simulink model "modelWithControllerAndBasicRobotDynamics"  (R2022a)
settings: Solver=VariableStepAuto  StartTime=0.0  StopTime=20  MaxStep=0.1  RelTol=1e-2  AbsTol=1e-2
model workspace (MAT data in the model file):
  jointLimits = [-2.94087978961  2.94087978961; -2.50454747661  0.759218224618; -2.94087978961  2.94087978961; -2.15548162621  1.3962634016; -5.06145483078  5.06145483078; -1.53588974176  2.40855436775; -3.99680398707  3.99680398707; 0  0.025; 0  0.025; -2.94087978961  2.94087978961; -2.50454747661  0.759218224618; -2.94087978961  2.94087978961; -2.15548162621  1.3962634016; -5.06145483078  5.06145483078; -1.53588974176  2.40855436775; -3.99680398707  3.99680398707; 0  0.025; 0  0.025]
values from neighbouring files (symbols this model uses):
  configSequence = [-0.501061022402 -0.485319444061 0.447530394494 -0.0261030910079 -0.440724306093 0.594332377665 0.0114553342542 0 0 0.712315437264 -1.59156502907 -0.483414164072 ... (126 elements, 18x7)]    [abbExampleRSTVariables.mat]    (also in abbSavedConfigs.mat)
  dq0 = [0 0 0 0 0 0 0 0 0 0 0 0 ... (18 elements, 18x1)]    [abbExampleRSTVariables.mat]
  q0 = [-0.501061022402 -0.485319444061 0.447530394494 -0.0261030910079 -0.440724306093 0.594332377665 0.0114553342542 0 0 0.712315437264 -1.59156502907 -0.483414164072 ... (18 elements, 18x1)]    [abbExampleRSTVariables.mat]
undefined symbols (not defined in the file or in its folder): robot
libraries: robotmaniplib x4, robotcorelib x1
settings Model: PauseTimes=3.1  Creator=The MathWorks, Inc.  LastModifiedBy=The MathWorks, Inc.
settings SolverCC: AlgebraicLoopSolver=TrustRegion
settings DebuggingCC: UnconnectedInputMsg=warning  UnconnectedOutputMsg=warning  UnconnectedLineMsg=warning  SFMachineParentedDataDiag=warning

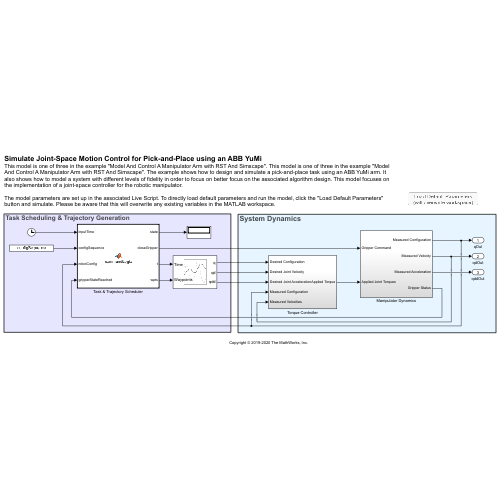
[thumbnail: Simulink's stored preview of the top-level diagram]
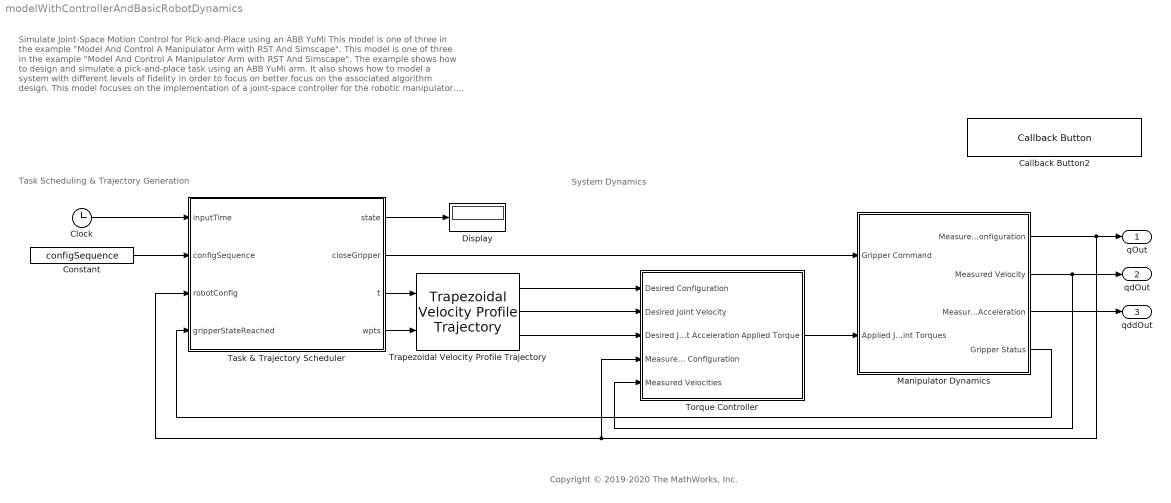
== system modelWithControllerAndBasicRobotDynamics ==
  note: Task Scheduling & Trajectory Generation
  note: System Dynamics
  note: Copyright © 2019-2020 The MathWorks, Inc.
  note: Simulate Joint-Space Motion Control for Pick-and-Place using an ABB YuMi
      | This model is one of three in the example "Model And Control A Manipulator Arm with RST And Simscape". This model is one of three in the example "Model And Control A Manipulator Arm with RST And Simscape". The example shows how to design and simulate a pick-and-place task using an ABB YuMi arm. It also shows how to model a system with different levels of fidelity in order to focus on better focus on the associated algorithm design. This model focuses on the implementation of a joint-space controller for the robotic manipulator.
      |
      | The model parameters are set up in the associated Live Script. To directly load default parameters and run the model, click the "Load Default Parameters" button and simulate. Please be aware that this will overwrite any existing variables in the MATLAB workspace.
  Callback Button2 : CallbackButton  ButtonText=Load Default Parameters (will overwrite workspace)
      settings: ClickFcn=|
      | robot = loadrobot('abbYumi', 'Gravity', [0 0 -9.81]);
      | load abbExampleRSTVariables.mat;
  Clock : Clock
  Constant : Constant  Value=configSequence
  Display : Display
  Manipulator Dynamics : Subsystem
  Task & Trajectory Scheduler : MATLAB Function  TreatAsAtomicUnit=on
  Torque Controller : Subsystem
  Trapezoidal Velocity Profile Trajectory : robotcorelib/Trapezoidal Velocity Profile Trajectory  WaypointSource=External  Waypoints=[ 0, -0.5, -1; 0, 0.5, 1 ]  NumParams=1  Parameter1=End Time  Parameter2=End Time  ParameterSource=Internal  PeakVelocity=[ 2; 2 ]  Acceleration=[ 1; 2 ]  EndTime=2  AccelTime=[ 1; 2 ]  SimulateUsing=Interpreted execution
      settings: SourceProductBaseCode=RO,NV,RR,UV
  qOut : Outport
  qdOut : Outport  Port=2
  qddOut : Outport  Port=3
  wires:
  Task & Trajectory Scheduler/3(t) -> Trapezoidal Velocity Profile Trajectory/1
  Task & Trajectory Scheduler/4(wpts) -> Trapezoidal Velocity Profile Trajectory/2
  Constant/1 -> Task & Trajectory Scheduler/2(configSequence)
  Task & Trajectory Scheduler/1(state) -> Display/1
  Trapezoidal Velocity Profile Trajectory/1 -> Torque Controller/1(Desired Configuration)
  Trapezoidal Velocity Profile Trajectory/2 -> Torque Controller/2(Desired Joint Velocity)
  Trapezoidal Velocity Profile Trajectory/3 -> Torque Controller/3(Desired Joint Acceleration)
  Manipulator Dynamics/1(Measured Configuration) -> Torque Controller/4(Measured Configuration), Task & Trajectory Scheduler/3(robotConfig), qOut/1
  Manipulator Dynamics/2(Measured Velocity) -> Torque Controller/5(Measured Velocities), qdOut/1
  Manipulator Dynamics/3(Measured Acceleration) -> qddOut/1
  Manipulator Dynamics/4(Gripper Status) -> Task & Trajectory Scheduler/4(gripperStateReached)
  Torque Controller/1(Applied Torque) -> Manipulator Dynamics/2(Applied Joint Torques)
  Task & Trajectory Scheduler/2(closeGripper) -> Manipulator Dynamics/1(Gripper Command)
  Clock/1 -> Task & Trajectory Scheduler/1(inputTime)

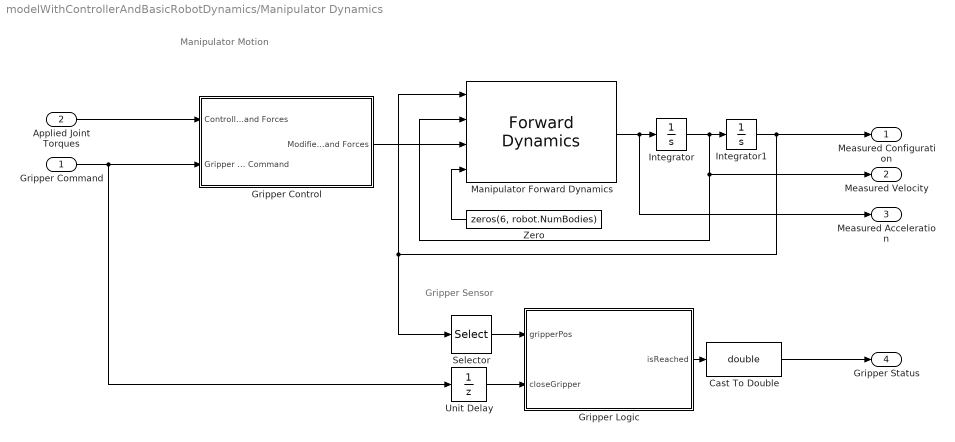
== system modelWithControllerAndBasicRobotDynamics/Manipulator Dynamics ==
  note: Gripper Sensor
  note: Manipulator Motion
  Gripper Command : Inport
  Applied Joint Torques : Inport  Port=2
  Cast To Double : DataTypeConversion  OutDataTypeStr=double  SaturateOnIntegerOverflow=off  RndMeth=Floor
  Gripper Control : Subsystem
  Gripper Logic : MATLAB Function  TreatAsAtomicUnit=on
  Integrator : Integrator  InitialCondition=dq0
  Integrator1 : Integrator  InitialCondition=q0  LimitOutput=on  UpperSaturationLimit=jointLimits(:,2)  LowerSaturationLimit=jointLimits(:,1)
  Manipulator Forward Dynamics : robotmaniplib/Forward Dynamics  RigidBodyTree=robot  SimulateUsing=Interpreted execution
  Selector : Selector  InputPortWidth=18  IndexOptions=Index vector (dialog)  Indices=[17 18]  OutputSizes=1
  Unit Delay : UnitDelay  SampleTime=-1  HasFrameUpgradeWarning=on
  Zero : Constant  Value=zeros(6, robot.NumBodies)  OutDataTypeStr=Inherit: Inherit via back propagation
  Measured Configuration : Outport  VectorParamsAs1DForOutWhenUnconnected=off
  Measured Velocity : Outport  Port=2  VectorParamsAs1DForOutWhenUnconnected=off
  Measured Acceleration : Outport  Port=3  VectorParamsAs1DForOutWhenUnconnected=off
  Gripper Status : Outport  Port=4  VectorParamsAs1DForOutWhenUnconnected=off
  wires:
  Zero/1 -> Manipulator Forward Dynamics/4
  Applied Joint Torques/1 -> Gripper Control/1(Controller Joint Torques and Forces)
  Integrator/1 -> Manipulator Forward Dynamics/2, Measured Velocity/1, Integrator1/1
  Manipulator Forward Dynamics/1 -> Integrator/1, Measured Acceleration/1
  Gripper Command/1 -> Unit Delay/1, Gripper Control/2(Gripper Close Command)
  Gripper Control/1(Modified Joint Torques and Forces) -> Manipulator Forward Dynamics/3
  Selector/1 -> Gripper Logic/1(gripperPos)
  Gripper Logic/1(isReached) -> Cast To Double/1
  Cast To Double/1 -> Gripper Status/1
  Unit Delay/1 -> Gripper Logic/2(closeGripper)
  Integrator1/1 -> Selector/1, Manipulator Forward Dynamics/1, Measured Configuration/1

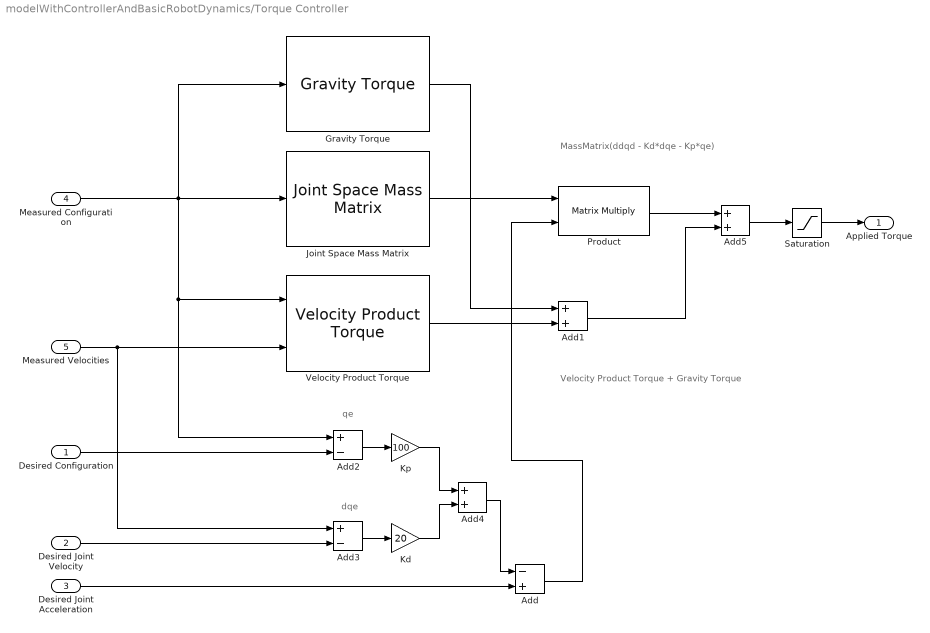
== system modelWithControllerAndBasicRobotDynamics/Torque Controller ==
  note: MassMatrix(ddqd - Kd*dqe - Kp*qe)
  note: Velocity Product Torque + Gravity Torque
  note: dqe
  note: qe
  Desired Configuration : Inport
  Desired Joint Velocity : Inport  Port=2
  Desired Joint Acceleration : Inport  Port=3
  Measured Configuration : Inport  Port=4
  Measured Velocities : Inport  Port=5
  Add : Sum  Inputs=-+
  Add1 : Sum
  Add2 : Sum  Inputs=+-
  Add3 : Sum  Inputs=+-
  Add4 : Sum
  Add5 : Sum
  Gravity Torque : robotmaniplib/Gravity Torque  RigidBodyTree=robot  SimulateUsing=Interpreted execution
  Joint Space Mass Matrix : robotmaniplib/Joint Space Mass Matrix  RigidBodyTree=robot  SimulateUsing=Interpreted execution
  Kd : Gain  Gain=20
  Kp : Gain  Gain=100
  Product : Product  Multiplication=Matrix(*)
  Saturation : Saturate  UpperLimit=100  LowerLimit=-100
  Velocity Product Torque : robotmaniplib/Velocity Product Torque  RigidBodyTree=robot  SimulateUsing=Interpreted execution
      settings: SourceProductBaseCode=RO
  Applied Torque : Outport  VectorParamsAs1DForOutWhenUnconnected=off
  wires:
  Saturation/1 -> Applied Torque/1
  Velocity Product Torque/1 -> Add1/2
  Gravity Torque/1 -> Add1/1
  Add1/1 -> Add5/2
  Product/1 -> Add5/1
  Add5/1 -> Saturation/1
  Kd/1 -> Add4/2
  Kp/1 -> Add4/1
  Add3/1 -> Kd/1
  Add2/1 -> Kp/1
  Add/1 -> Product/2
  Add4/1 -> Add/1
  Measured Velocities/1 -> Velocity Product Torque/2, Add3/1
  Measured Configuration/1 -> Add2/1, Velocity Product Torque/1, Gravity Torque/1, Joint Space Mass Matrix/1
  Joint Space Mass Matrix/1 -> Product/1
  Desired Configuration/1 -> Add2/2
  Desired Joint Velocity/1 -> Add3/2
  Desired Joint Acceleration/1 -> Add/2

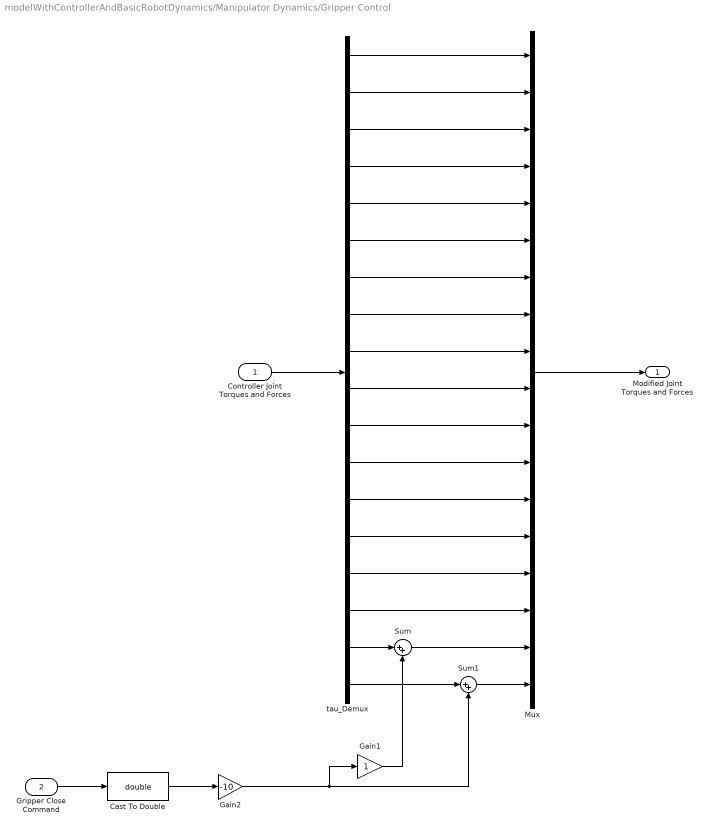
== system modelWithControllerAndBasicRobotDynamics/Manipulator Dynamics/Gripper Control ==
  Controller Joint Torques and Forces : Inport
  Gripper Close Command : Inport  Port=2
  Cast To Double : DataTypeConversion  OutDataTypeStr=double  SaturateOnIntegerOverflow=off  RndMeth=Floor
  Gain1 : Gain
  Gain2 : Gain  Gain=-10
  Mux : Mux  Inputs=18
  Sum : Sum  Inputs=|++
  Sum1 : Sum  Inputs=|++
  tau_Demux : Demux  Outputs=18
  Modified Joint Torques and Forces : Outport
  wires:
  Mux/1 -> Modified Joint Torques and Forces/1
  tau_Demux/5 -> Mux/5
  Gripper Close Command/1 -> Cast To Double/1
  tau_Demux/10 -> Mux/10
  tau_Demux/7 -> Mux/7
  tau_Demux/9 -> Mux/9
  Controller Joint Torques and Forces/1 -> tau_Demux/1
  tau_Demux/4 -> Mux/4
  tau_Demux/2 -> Mux/2
  tau_Demux/14 -> Mux/14
  tau_Demux/3 -> Mux/3
  Cast To Double/1 -> Gain2/1
  tau_Demux/6 -> Mux/6
  tau_Demux/13 -> Mux/13
  tau_Demux/15 -> Mux/15
  tau_Demux/8 -> Mux/8
  tau_Demux/16 -> Mux/16
  Gain2/1 -> Sum1/2, Gain1/1
  tau_Demux/12 -> Mux/12
  tau_Demux/11 -> Mux/11
  tau_Demux/1 -> Mux/1
  tau_Demux/17 -> Sum/1
  tau_Demux/18 -> Sum1/1
  Gain1/1 -> Sum/2
  Sum/1 -> Mux/17
  Sum1/1 -> Mux/18

== matlab function modelWithControllerAndBasicRobotDynamics/Manipulator Dynamics/Gripper Logic ==
  data: gripperPos input; closeGripper input; isReached output
function isReached = isGripperStateReached(gripperPos, closeGripper)

    isReached = false;

    % Define key values
    posTgtThreshold = 0.01;
    openValue = 0.025;
    closeValue = 0;
    
    if closeGripper
        gripperTarget = closeValue;
    else
        gripperTarget = openValue;
    end
    
    % Check if the gripper joints have reached their open target
    diffWpts = abs(gripperPos - [gripperTarget; gripperTarget]);
    posErrorStatus = diffWpts < posTgtThreshold;
    
    if all(posErrorStatus)
        isReached = true;
    end
    
end

== matlab function modelWithControllerAndBasicRobotDynamics/Task & Trajectory Scheduler ==
  settings: updateMethod=DISCRETE
  data: inputTime input; configSequence input; state output; closeGripper output; robotConfig input; t output; wpts output; gripperStateReached input
function [state, closeGripper, t, wpts] = commandLogic(inputTime, configSequence, robotConfig, gripperStateReached)

persistent motionState
persistent resetTimeValue

% Set some variables
posTgtThreshold = 0.015;

% Initialize persistent variables
if isempty(motionState)
    motionState = 0;
end
if isempty(resetTimeValue)
    resetTimeValue = 0;
end

% Output the state and time
state = motionState;
t = inputTime - resetTimeValue;

% Initialize outputs to starting state
wpts = configSequence(:,1:2);
closeGripper = false;

switch motionState
    case 1
        % Grasp: Move from approach to grasp & open the gripper
        wpts = configSequence(:,2:3);
        closeGripper = false;
    case 2
        % Close the gripper
        wpts = [configSequence(:,3) configSequence(:,3)];
        closeGripper = true;
    case 3
        % Depart grasp
        wpts = configSequence(:,3:4);
        closeGripper = true;
    case 4
        % Move to place approach
        wpts = configSequence(:,4:5);
        closeGripper = true;
    case 5
        % Move to place
        wpts = configSequence(:,5:6);
        closeGripper = true;
    case 6
        % Open the gripper
        wpts = [configSequence(:,6) configSequence(:,6)];
        closeGripper = false;
    case 7
        % Depart place
        wpts = configSequence(:,6:7);
        closeGripper = false;
    case 8
        % Cycle to grasp approach
        wpts = configSequence(:,[7 2]);
        closeGripper = false;
end
   
% Get the current status
trajEndConfigReached = endStateReached(robotConfig, wpts, posTgtThreshold);

% Advance the state and reset time as needed
if trajEndConfigReached && gripperStateReached
    % Advance the state and reset the time
    motionState = mod(motionState, 7) + 1;
    resetTimeValue = inputTime;
end

end

function isReached = endStateReached(config, wpts, tgtThreshold)
    
    % Initialize output
    isReached = false;
    
    % Mark config states that are specific to gripper
    armStateExclGripperIdx = 10:16;
    
    %Extract the arm that matters and then ignore the gripper position
    armConfig = config(armStateExclGripperIdx,:);
    armTarget = wpts(armStateExclGripperIdx,2);
    
    % Check if the arm states match the target waypoints
    diffWpts = zeros(length(armStateExclGripperIdx),1);
    diffWpts(:,:) = abs(armConfig - armTarget);
    errorStatus = diffWpts < tgtThreshold;
    if all(errorStatus)
        isReached = true;
    end
end
